simulink model "RW_Time_Delay_Analysis_mdl_cont_codeversion"  (R2025b)
settings: Solver=VariableStepAuto  StartTime=0.0  StopTime=20  RelTol=1e-3
values from neighbouring files (symbols this model uses):
  Kd = 0.95    [RW_Time_Delay_Analysis.m]    (also in RW_Time_Delay_Analysis_Simulink_Params.m; RW_Time_Delay_Analysis_new_implementation.m)
  Ki = 0.1    [RW_Time_Delay_Analysis.m]    (also in RW_Time_Delay_Analysis_Simulink_Params.m; RW_Time_Delay_Analysis_new_implementation.m)
  Kp = 0.8    [RW_Time_Delay_Analysis.m]    (also in RW_Time_Delay_Analysis_Simulink_Params.m; RW_Time_Delay_Analysis_new_implementation.m)
settings Model: Creator=barinmoghimi  LastModifiedBy=barinmoghimi

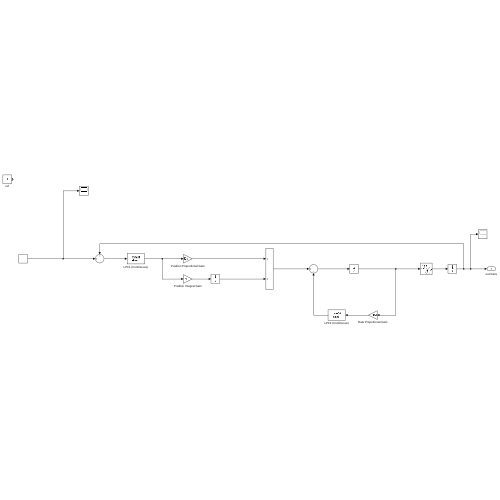
[thumbnail: Simulink's stored preview of the top-level diagram]
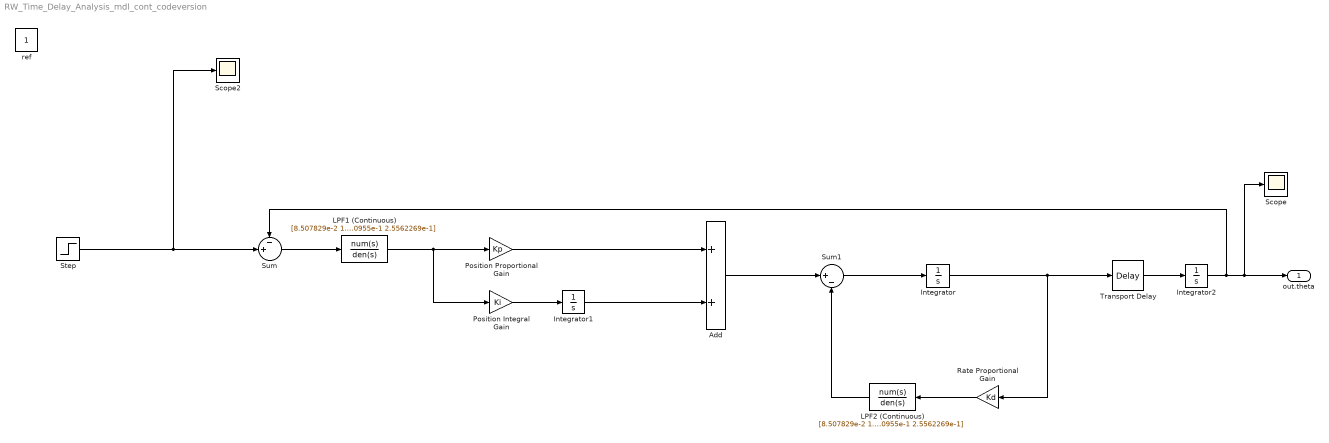
== system RW_Time_Delay_Analysis_mdl_cont_codeversion ==
  Add : Sum
  Integrator : Integrator
  Integrator1 : Integrator
  Integrator2 : Integrator
  LPF1 (Continuous) : TransferFcn  Numerator=[8.507829e-2 1.7015657e-1 8.50782e-2]  Denominator=[1.0e+0 -9.1530955e-1 2.5562269e-1]
  LPF2 (Continuous) : TransferFcn  Numerator=[8.507829e-2 1.7015657e-1 8.50782e-2]  Denominator=[1.0e+0 -9.1530955e-1 2.5562269e-1]
  Position Integral Gain : Gain  Gain=Ki
  Position Proportional Gain : Gain  Gain=Kp
  Rate Proportional Gain : Gain  Gain=Kd
  Scope : Scope
      settings: ActiveDisplayYMinimum=-43818.650588918434  ActiveDisplayYMaximum=8148.19694969838
  Scope2 : Scope
      settings: ActiveDisplayYMinimum=-0.12499999999999997  ActiveDisplayYMaximum=1.125  DataLoggingVariableName=ScopeData2
  Step : Step  SampleTime=0
  Sum : Sum  Inputs=-+|
  Sum1 : Sum  Inputs=|+-
  Transport Delay : TransportDelay  DelayTime=.3
  ref : Constant
  out.theta : Outport
  wires:
  Position Proportional Gain/1 -> Add/1
  Step/1 -> Scope2/1, Sum/2
  Sum/1 -> LPF1 (Continuous)/1
  LPF1 (Continuous)/1 -> Position Integral Gain/1, Position Proportional Gain/1
  Position Integral Gain/1 -> Integrator1/1
  Integrator1/1 -> Add/2
  Add/1 -> Sum1/1
  Sum1/1 -> Integrator/1
  Rate Proportional Gain/1 -> LPF2 (Continuous)/1
  LPF2 (Continuous)/1 -> Sum1/2
  Integrator/1 -> Rate Proportional Gain/1, Transport Delay/1
  Transport Delay/1 -> Integrator2/1
  Integrator2/1 -> Scope/1, out.theta/1, Sum/1
